simulink model "im_model_exercise_version"  (Simulink 7.4)
settings: Solver=ode45  StartTime=0.0  StopTime=1  MaxStep=1e-3  RelTol=1e-5
InitFcn:
  | im_data
values from neighbouring files (symbols this model uses):
  In = 5.1    [im_data.m]
  Omegae = 2*pi*fn    (= 314.159265359)    [im_data.m]
  Un = 220    [im_data.m]
Description:
  | Induction machine model as in Kaz. p 34
  | 
  | Note errors in (1.128) for rotor equations (Lm->Lr for some terms)!
settings Model: Creator=Michael M. Bech  LastModifiedBy=klu  ExtModeTrigMode=oneshot  ExtModeArmWhenConnect=off
settings DataIOCC: LimitDataPoints=off
settings OptimizationCC: BlockReduction=off  BooleanDataType=off  InlineInvariantSignals=on  InitFltsAndDblsToZero=on
settings DebuggingCC: SaveWithParameterizedLinksMsg=none  SignalResolutionControl=TryResolveAllWithWarning  SolverPrmCheckMsg=none  MultiTaskDSMMsg=warning  MultiTaskCondExecSysMsg=none  StrictBusMsg=None
settings HardwareCC: TargetUnknown=on
settings RTWCC: IncludeERTFirstTime=on
settings GRTTargetCC: TargetFcnLib=ansi_tfl_tmw.mat

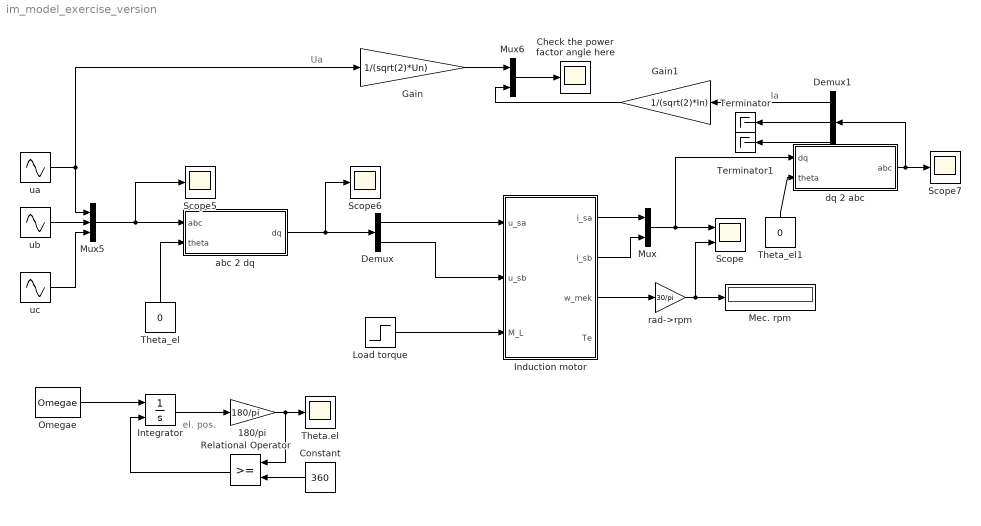
== system im_model_exercise_version ==
  note: el. pos.
  note: Ua
  note: Ia
  180/pi : Gain  Gain=180/pi  ParameterDataType=sfix(16)  ParameterScaling=2^0  OutDataType=sfix(16)  OutScaling=2^0
  Check the power factor angle here : Scope
      settings: SaveName=ScopeData9
  Constant : Constant  Value=360  OutDataType=sfix(16)  OutScaling=2^0
  Demux : Demux  Outputs=2
  Demux1 : Demux  Outputs=3
  Gain : Gain  Gain=1/(sqrt(2)*Un)  ParameterDataType=sfix(16)  ParameterScaling=2^0  OutDataType=sfix(16)  OutScaling=2^0
  Gain1 : Gain  Gain=1/(sqrt(2)*In)  ParameterDataType=sfix(16)  ParameterScaling=2^0  OutDataType=sfix(16)  OutScaling=2^0
  Induction motor : Subsystem
  Integrator : Integrator  ExternalReset=rising
  Load torque : Step  Time=0.25  After=14.6912  SampleTime=0
  Mec. rpm : Display
  Mux : Mux  Inputs=2
  Mux5 : Mux  Inputs=3
  Mux6 : Mux  Inputs=2
  Omegae : Constant  Value=Omegae  OutDataType=sfix(16)  OutScaling=2^0
  Relational Operator : RelationalOperator  LogicOutDataTypeMode=boolean  OutDataTypeStr=boolean
  Scope : Scope  NumInputPorts=2
      settings: TimeRange=0.5  YMin=-40~0  YMax=40~1750
  Scope5 : Scope
      settings: SaveName=ScopeData5
  Scope6 : Scope
      settings: SaveName=ScopeData7
  Scope7 : Scope
      settings: SaveName=ScopeData8
  Terminator : Terminator
  Terminator1 : Terminator
  Theta.el : Scope
      settings: YMin=-225  YMax=225  SaveName=ScopeData6
  Theta_el : Constant  Value=0  OutDataType=sfix(16)  OutScaling=2^0
  Theta_el1 : Constant  Value=0  OutDataType=sfix(16)  OutScaling=2^0
  abc 2 dq : Subsystem
  dq 2 abc : Subsystem
  rad->rpm : Gain  Gain=30/pi  ParameterDataType=sfix(16)  ParameterScaling=2^0  OutDataType=sfix(16)  OutScaling=2^0  SaturateOnIntegerOverflow=on  OutDataTypeStr=Inherit: Same as input  ParamDataTypeStr=Inherit: Same as input
  ua : Sin  Amplitude=sqrt(2)*Un  Bias=0  Frequency=Omegae  Phase=pi/2  Samples=10  SampleTime=0  Offset=0
  ub : Sin  Amplitude=sqrt(2)*Un  Bias=0  Frequency=Omegae  Phase=pi/2-120/180*pi  Samples=10  SampleTime=0  Offset=0
  uc : Sin  Amplitude=sqrt(2)*Un  Bias=0  Frequency=Omegae  Phase=pi/2-240/180*pi  Samples=10  SampleTime=0  Offset=0
  wires:
  Induction motor/1(i_sa) -> Mux/1
  Induction motor/2(i_sb) -> Mux/2
  Mux/1 -> Scope/1, dq 2 abc/1(dq)
  Induction motor/3(w_mek) -> rad->rpm/1
  rad->rpm/1 -> Mec. rpm/1, Scope/2
  abc 2 dq/1(dq) -> Demux/1, Scope6/1
  Demux/2 -> Induction motor/2(u_sb)
  ua/1 -> Mux5/1, Gain/1
  uc/1 -> Mux5/3
  ub/1 -> Mux5/2
  Mux5/1 -> abc 2 dq/1(abc), Scope5/1
  Integrator/1 -> 180/pi/1
  180/pi/1 -> Theta.el/1, Relational Operator/1
  Constant/1 -> Relational Operator/2
  Relational Operator/1 -> Integrator/2
  Load torque/1 -> Induction motor/3(M_L)
  Omegae/1 -> Integrator/1
  Theta_el/1 -> abc 2 dq/2(theta)
  Demux/1 -> Induction motor/1(u_sa)
  Theta_el1/1 -> dq 2 abc/2(theta)
  dq 2 abc/1(abc) -> Scope7/1, Demux1/1
  Mux6/1 -> Check the power factor angle here/1
  Gain/1 -> Mux6/1
  Demux1/2 -> Terminator/1
  Demux1/3 -> Terminator1/1
  Demux1/1 -> Gain1/1
  Gain1/1 -> Mux6/2

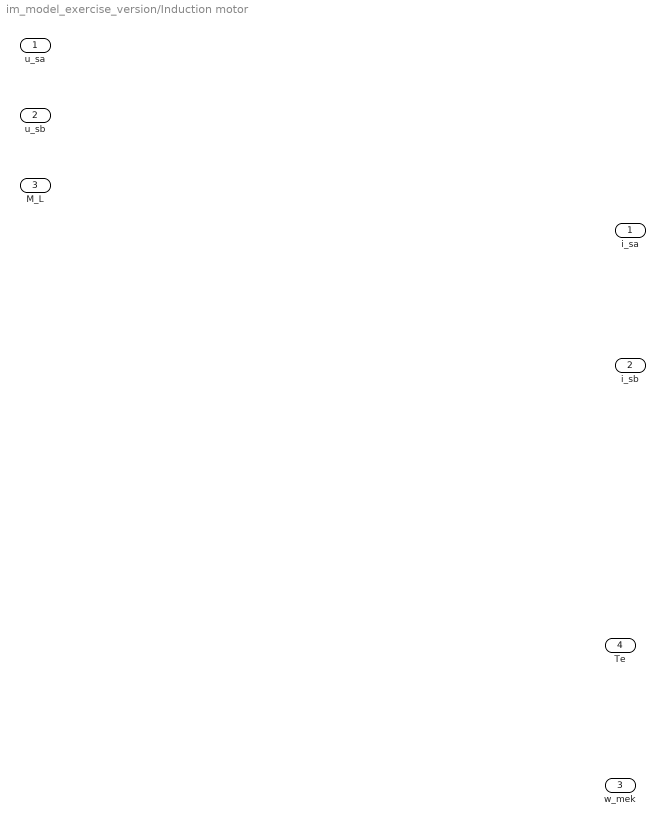
== system im_model_exercise_version/Induction motor ==
  u_sa : Inport  OutDataType=sfix(16)  OutScaling=2^0
  u_sb : Inport  Port=2  OutDataType=sfix(16)  OutScaling=2^0
  M_L : Inport  Port=3  OutDataType=sfix(16)  OutScaling=2^0
  i_sa : Outport  OutDataType=sfix(16)  OutScaling=2^0
  i_sb : Outport  Port=2  OutDataType=sfix(16)  OutScaling=2^0
  w_mek : Outport  Port=3  OutDataType=sfix(16)  OutScaling=2^0
  Te : Outport  Port=4  OutDataType=sfix(16)  OutScaling=2^0

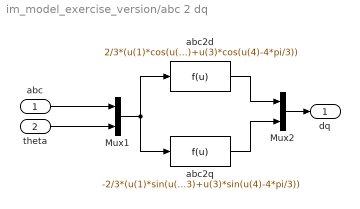
== system im_model_exercise_version/abc 2 dq ==
  abc : Inport  OutDataType=sfix(16)  OutScaling=2^0
  theta : Inport  Port=2  OutDataType=sfix(16)  OutScaling=2^0
  Mux1 : Mux  Inputs=2
  Mux2 : Mux  Inputs=2
  abc2d : Fcn  Expr=2/3*(u(1)*cos(u(4))+u(2)*cos(u(4)-2*pi/3)+u(3)*cos(u(4)-4*pi/3))
  abc2q : Fcn  Expr=-2/3*(u(1)*sin(u(4))+u(2)*sin(u(4)-2*pi/3)+u(3)*sin(u(4)-4*pi/3))
  dq : Outport  OutDataType=sfix(16)  OutScaling=2^0
  wires:
  abc/1 -> Mux1/1
  theta/1 -> Mux1/2
  Mux1/1 -> abc2d/1, abc2q/1
  abc2d/1 -> Mux2/1
  abc2q/1 -> Mux2/2
  Mux2/1 -> dq/1

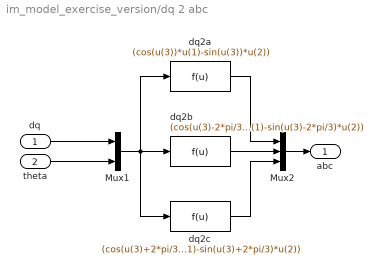
== system im_model_exercise_version/dq 2 abc ==
  dq : Inport  OutDataType=sfix(16)  OutScaling=2^0
  theta : Inport  Port=2  OutDataType=sfix(16)  OutScaling=2^0
  Mux1 : Mux  Inputs=2
  Mux2 : Mux  Inputs=3
  dq2a : Fcn  Expr=(cos(u(3))*u(1)-sin(u(3))*u(2))
  dq2b : Fcn  Expr=(cos(u(3)-2*pi/3)*u(1)-sin(u(3)-2*pi/3)*u(2))
  dq2c : Fcn  Expr=(cos(u(3)+2*pi/3)*u(1)-sin(u(3)+2*pi/3)*u(2))
  abc : Outport  OutDataType=sfix(16)  OutScaling=2^0
  wires:
  Mux2/1 -> abc/1
  dq2b/1 -> Mux2/2
  dq2a/1 -> Mux2/1
  Mux1/1 -> dq2a/1, dq2c/1, dq2b/1
  theta/1 -> Mux1/2
  dq/1 -> Mux1/1
  dq2c/1 -> Mux2/3
